simulink model "TST_AdvancedStateflowLoops4"  (Simulink 10.0)
settings: Solver=FixedStepDiscrete  StartTime=0.0  StopTime=10.0  FixedStep=0.02  RelTol=1e-3  EnableMultiTasking=on
settings Model: Creator=kharthforeign  LastModifiedBy=unknown
settings DataIOCC: LimitDataPoints=on  SignalLoggingSaveFormat=ModelDataLogs  SaveOutput=off  SignalLogging=off  SaveTime=off
settings OptimizationCC: BlockReduction=off  ConditionallyExecuteInputs=off  OptimizeBlockIOStorage=off  BufferReuse=off  GlobalBufferReuse=off  ExpressionFolding=off  ExpressionDepthLimit=2147483647  LocalBlockOutputs=off  InitFltsAndDblsToZero=on  OptimizeDataStoreBuffers=off  BusAssignmentInplaceUpdate=off
settings DebuggingCC: SolverPrmCheckMsg=warning  FcnCallInpInsideContextMsg=warning  StateNameClashWarn=warning
settings GRTTargetCC: GeneratePreprocessorConditionals=Disable all
settings ConfigComp: CovExternalEMLEnable=off

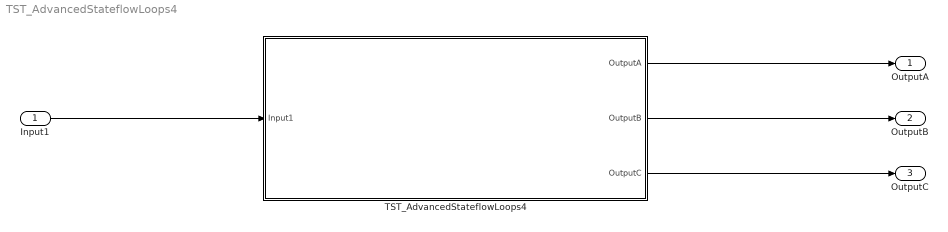
== system TST_AdvancedStateflowLoops4 ==
  Input1 : Inport  OutDataTypeStr=uint32  BusOutputAsStruct=on
  TST_AdvancedStateflowLoops4 : Subsystem  TreatAsAtomicUnit=on
  OutputA : Outport  OutDataTypeStr=double  PortDimensions=1
  OutputB : Outport  Port=2  OutDataTypeStr=double  PortDimensions=1
  OutputC : Outport  Port=3  OutDataTypeStr=double  PortDimensions=1
  wires:
  Input1/1 -> TST_AdvancedStateflowLoops4/1(Input1)
  TST_AdvancedStateflowLoops4/1(OutputA) -> OutputA/1
  TST_AdvancedStateflowLoops4/2(OutputB) -> OutputB/1
  TST_AdvancedStateflowLoops4/3(OutputC) -> OutputC/1

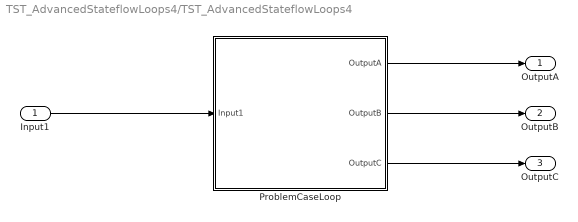
== system TST_AdvancedStateflowLoops4/TST_AdvancedStateflowLoops4 ==
  Input1 : Inport  OutDataTypeStr=uint32  BusOutputAsStruct=on
  ProblemCaseLoop : Stateflow chart  TreatAsAtomicUnit=on
  OutputA : Outport  OutDataTypeStr=double  PortDimensions=1
  OutputB : Outport  Port=2  OutDataTypeStr=double  PortDimensions=1
  OutputC : Outport  Port=3  OutDataTypeStr=double  PortDimensions=1
  wires:
  ProblemCaseLoop/1(OutputA) -> OutputA/1
  ProblemCaseLoop/2(OutputB) -> OutputB/1
  ProblemCaseLoop/3(OutputC) -> OutputC/1
  Input1/1 -> ProblemCaseLoop/1(Input1)

== stateflow chart TST_AdvancedStateflowLoops4/ProblemCaseLoop ==
  note: This flowgraph shows a current problem case for the code-generator,
      | where the first vertex of the loop is not the one with the loop condition
  note: #2
  note: #1
  note: #3
  note: #5
  note: #4
  (default) -> (junction 18)
  (junction 19) -> (junction 18) : {OutputA += 2.0}
  (junction 18) -> (junction 21) : {OutputA = 1.0}
  (junction 21) -> (junction 19) [order 1] : [A]
  (junction 21) -> (junction 20) [order 2] : [B]
  (junction 21) -> (junction 22) [order 3]
  data: Input1 input uint32; OutputA output double =1; OutputB output double =2; OutputC output double =3; Local local uint32 =0; A local boolean; B local boolean; C local boolean; D local boolean
